simulink model "model_sim_classic"  (R2024b)
settings: Solver=FixedStepAuto  StartTime=0.0  StopTime=tsim  FixedStep=T  RelTol=1e-3
values from neighbouring files (symbols this model uses):
  Kd = 1.5    [gains.m]
  Ki = [0.01, 0.282]    [gains.m]
  Kp = [2, 9.46]    [gains.m]
undefined symbols (not defined in the file or in its folder): T
libraries: slpidlib x1
settings Model: Creator=usuario  LastModifiedBy=usuario
settings DataIOCC: ReturnWorkspaceOutputs=off  TimeSaveName=t
settings RTWCC: GPUComputeCapability=3.5

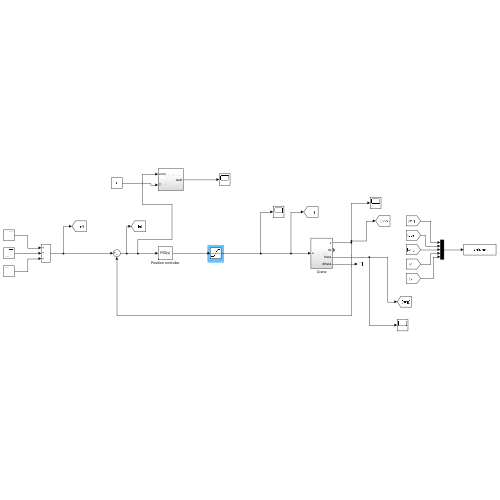
[thumbnail: Simulink's stored preview of the top-level diagram]
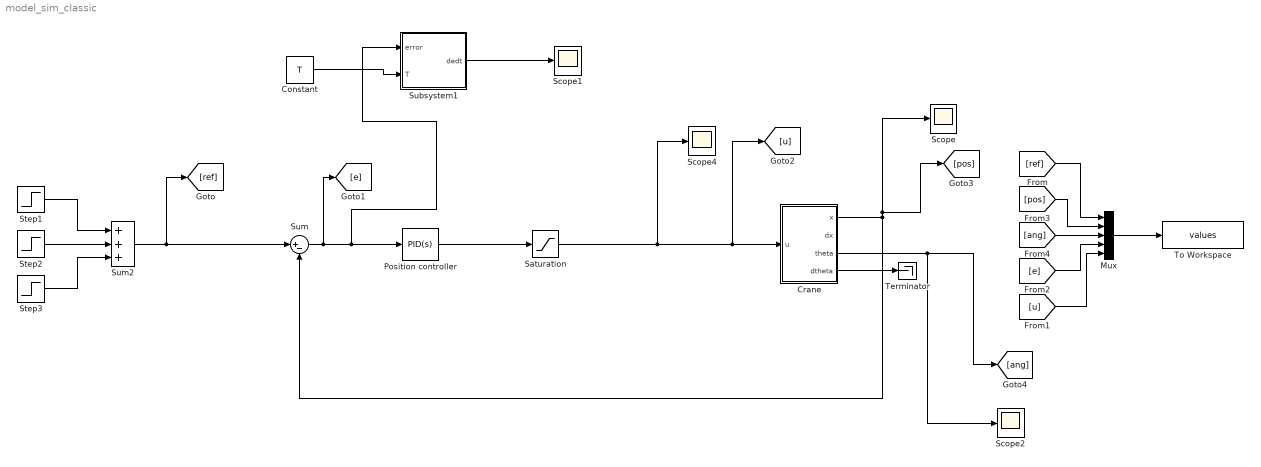
== system model_sim_classic ==
  Constant : Constant  Value=T
  Crane : Subsystem
  Mux : Mux  Inputs=5
  Position controller : slpidlib/PID Controller  Controller=PID  Form=Parallel  TimeDomain=Continuous-time  UseExternalTs=off  SampleTime=-1  IntegratorMethod=Forward Euler  FilterMethod=Forward Euler  ControllerParametersSource=internal  P=Kp(1)  I=Ki(1)  UseKiTs=off  D=Kd  UseExternalDerivativeSource=off  N=100  UseFilter=on  TunerSelectOption=Transfer Function Based (PID Tuner App)  InitialConditionSource=internal  InitialConditionForIntegrator=0  InitialConditionForFilter=0  DifferentiatorICPrevScaledInput=0  ExternalReset=none  TrackingMode=off  Kt=1  LimitOutput=off  SatLimitsSource=internal  UpperSaturationLimit=30  LowerSaturationLimit=-30  LinearizeAsGain=on  AntiWindupMode=none  Kb=1  LimitIntegrator=off  UpperIntegratorSaturationLimit=inf  LowerIntegratorSaturationLimit=-inf  POutMin=[]  POutMax=[]  IOutMin=[]  IOutMax=[]  DOutMin=[]  DOutMax=[]  NOutMin=[]  NOutMax=[]  SumOutMin=[]  SumOutMax=[]  SaturationOutMin=[]  SaturationOutMax=[]  PParamMin=[]  PParamMax=[]  IParamMin=[]  IParamMax=[]  DParamMin=[]  DParamMax=[]  NParamMin=[]  NParamMax=[]  KbParamMin=[]  KbParamMax=[]  KtParamMin=[]  KtParamMax=[]  KbOutMin=[]  KbOutMax=[]  KtOutMin=[]  KtOutMax=[]  IntegratorOutMin=[]  IntegratorOutMax=[]  FilterOutMin=[]  FilterOutMax=[]  SumI1OutMin=[]  SumI1OutMax=[]  SumI2OutMin=[]  SumI2OutMax=[]  SumI3OutMin=[]  SumI3OutMax=[]  SumI4OutMin=[]  SumI4OutMax=[]  SumDOutMin=[]  SumDOutMax=[]  DifferentiatorOutMin=[]  DifferentiatorOutMax=[]  FilterDiffOutCoefMin=[]  FilterDiffOutCoefMax=[]  ReciprocalOutMin=[]  ReciprocalOutMax=[]  SumDenOutMin=[]  SumDenOutMax=[]  SumNumOutMin=[]  SumNumOutMax=[]  DivideOutMin=[]  DivideOutMax=[]  UdiffTsProdOutMin=[]  UdiffTsProdOutMax=[]  NTsProdOutMin=[]  NTsProdOutMax=[]  UintegralTsProdOutMin=[]  UintegralTsProdOutMax=[]  UngainTsProdOutMin=[]  UngainTsProdOutMax=[]  ClampingZeroOutDataTypeStr=Inherit: Inherit via back propagation  ClampingZeroOutMin=[]  ClampingZeroOutMax=[]  FilterDenConstantOutDataTypeStr=Inherit: Inherit via back propagation  FilterDenConstantOutMin=[]  FilterDenConstantOutMax=[]  PCopyOutDataTypeStr=Inherit: Inherit via back propagation  PCopyOutMin=[]  PCopyOutMax=[]  NCopyOutDataTypeStr=Inherit: Inherit via back propagation  NCopyOutMin=[]  NCopyOutMax=[]  IntegratorContinuousStateAttributes=''  IntegratorStateMustResolveToSignalObject=off  IntegratorRTWStateStorageClass=Auto  FilterContinuousStateAttributes=''  FilterStateMustResolveToSignalObject=off  FilterRTWStateStorageClass=Auto  ParallelPVariant=InternalParameters  IdealPVariant=Disabled  IVariant=InternalParameters  DVariant=InternalParameters  IntegratorVariant=Continuous  SatVariant=Disabled  AWVariant=Passthrough  PCopyVariant=Disabled  TRVariant=Disabled  FdbkBlocksVariant=Forward  IdealPFdbkVariant=Disabled  SatFdbkVariant=Disabled  DerivativeFilterVariant=ContFilter  NVariant=InternalParameters  NCopyVariant=Disabled  FilterICVariant=InternalICsFilter  IntegratorICVariant=InternalICs  ExternalResetVariant=Disabled  TRSumVariant=Passthrough  SumFdbkVariant=Disabled  SumVariant=Sum_PID  TsampFilterVariant=InternalTs  TsampNgainVariant=Passthrough  TsampIntegralVariant=Disabled_SignalSpec  ExternalSaturationOutDataTypeStr=Inherit: Same as second input  DerivativeSourceVariant=ErrorSignal  PreIntVariant=InternalPreInt
  Saturation : Saturate  UpperLimit=30  LowerLimit=-30
  Scope{,1..2,4} (4 alike) : Scope
  Step1 : Step  Time=0  After=0.6  SampleTime=0
  Step2 : Step  Time=15  After=0.4  SampleTime=0
  Step3 : Step  Time=30  After=-0.7  SampleTime=0
  Subsystem1 : Subsystem
  Sum : Sum  Inputs=|+-
  Sum2 : Sum  Inputs=+++
  Terminator : Terminator
  To Workspace : ToWorkspace  VariableName=values  SaveFormat=Structure  SampleTime=-1
  wires:
  Mux/1 -> To Workspace/1
  Crane/1(x) -> [pos], Scope/1, Sum/2
  Sum/1 -> [e], Subsystem1/1(error), Position controller/1
  Crane/4(dtheta) -> Terminator/1
  [ref] -> Mux/1
  [pos] -> Mux/2
  [ang] -> Mux/3
  [e] -> Mux/4
  [u] -> Mux/5
  Constant/1 -> Subsystem1/2(T)
  Subsystem1/1(dedt) -> Scope1/1
  Step1/1 -> Sum2/1
  Step3/1 -> Sum2/3
  Step2/1 -> Sum2/2
  Crane/3(theta) -> [ang], Scope2/1
  Sum2/1 -> Sum/1, [ref]
  Position controller/1 -> Saturation/1
  Saturation/1 -> Scope4/1, [u], Crane/1(u)

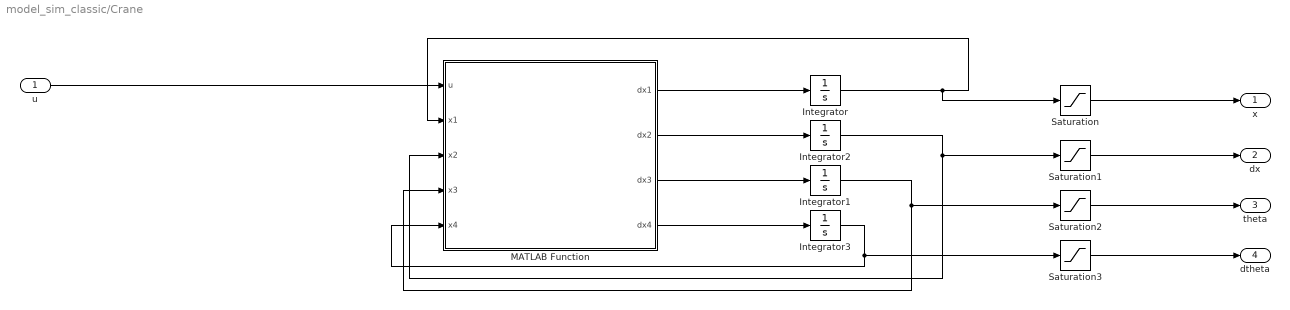
== system model_sim_classic/Crane ==
  u : Inport
  Integrator : Integrator  InitialCondition=0.002
  Integrator1 : Integrator  InitialCondition=0.001
  Integrator2 : Integrator
  Integrator3 : Integrator
  MATLAB Function : MATLAB Function  TreatAsAtomicUnit=on
  Saturation : Saturate  UpperLimit=3  LowerLimit=-3
  Saturation1 : Saturate  UpperLimit=5  LowerLimit=-5
  Saturation2 : Saturate  UpperLimit=pi/12  LowerLimit=-pi/12
  Saturation3 : Saturate  UpperLimit=pi/4  LowerLimit=-pi/4
  x : Outport
  dx : Outport  Port=2
  theta : Outport  Port=3
  dtheta : Outport  Port=4
  wires:
  MATLAB Function/2(dx2) -> Integrator2/1
  Integrator/1 -> Saturation/1, MATLAB Function/2(x1)
  Integrator2/1 -> MATLAB Function/3(x2), Saturation1/1
  MATLAB Function/4(dx4) -> Integrator3/1
  MATLAB Function/1(dx1) -> Integrator/1
  MATLAB Function/3(dx3) -> Integrator1/1
  Integrator3/1 -> MATLAB Function/5(x4), Saturation3/1
  Integrator1/1 -> Saturation2/1, MATLAB Function/4(x3)
  u/1 -> MATLAB Function/1(u)
  Saturation/1 -> x/1
  Saturation1/1 -> dx/1
  Saturation2/1 -> theta/1
  Saturation3/1 -> dtheta/1

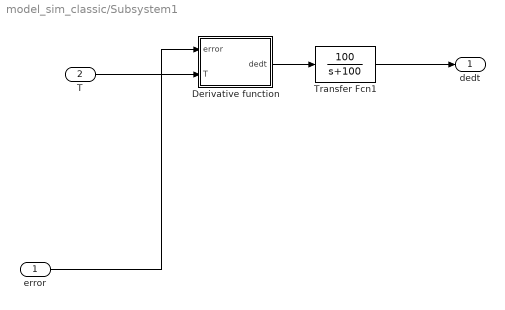
== system model_sim_classic/Subsystem1 ==
  error : Inport
  T : Inport  Port=2
  Derivative function : MATLAB Function  TreatAsAtomicUnit=on  SystemSampleTime=T
  Transfer Fcn1 : TransferFcn  Numerator=100  Denominator=[1 100]
  dedt : Outport
  wires:
  error/1 -> Derivative function/1(error)
  T/1 -> Derivative function/2(T)
  Derivative function/1(dedt) -> Transfer Fcn1/1
  Transfer Fcn1/1 -> dedt/1

== matlab function model_sim_classic/Subsystem1/Derivative function ==
  data: error input; dedt output; T input
function dedt = fcn(error, T)
    persistent p_error;
    if isempty(p_error)
        p_error = error;
    end
    dedt = (error - p_error)/T;
    p_error = error;
end

== matlab function model_sim_classic/Crane/MATLAB Function ==
  data: u input; dx1 output; x1 input; x2 input; x3 input; x4 input; dx2 output; dx3 output; dx4 output
function [dx1,dx2,dx3,dx4] = plant_model(u,x1,x2,x3,x4)
M = 10;g=9.8;m=5;l=1;mu=0.3;
q = [x1;x2;x3;x4];
a11 = -mu/(M+m*sin(x3)^2); a12 = m*g*cos(x3)*sin(x3)/((M+m*sin(x3)^2)*x3);
a13 = m*l*x4*sin(x3)/(M+m*sin(x3)^2); a21 = mu*cos(x3)/(l*(M+m*sin(x3)^2));
a22 = -(M+m)*g*sin(x3)/(l*x3*(M+m*sin(x3)^2)); a23=-m*x4*sin(x3)*cos(x3)/(M+m*sin(x3)^2);
b1 = 1/(M+m*sin(x3)^2); b2 = -cos(x3)/(l*(M+m*sin(x3)^2));
A = [0 1 0 0;0 a11 a12 a13;0 0 0 1;0 a21 a22 a23];
B = [0;b1;0;b2];

dq = A*q + B*u;
dx1 = dq(1);
dx2 = dq(2);
dx3 = dq(3);
dx4 = dq(4);
